simulink model "Drehteller"  (R2021a)
settings: Solver=VariableStepAuto  StartTime=0.0  StopTime=10.0  RelTol=1e-3
values from neighbouring files (symbols this model uses):
  A = 5    [Parametriesierung.m]
  I = 0.5    [Parametriesierung.m]
  igetr = 1080    [Parametriesierung.m]
  K = 8    [Parametriesierung.m]
  MRK = 1    [Parametriesierung.m]
  PHI = 0.001    [Parametriesierung.m]
  Ra = 40    [Parametriesierung.m]
  U = 24    [Parametriesierung.m]
settings Model: Creator=Oceaner  LastModifiedBy=Oceaner

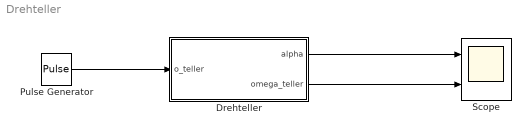
== system Drehteller ==
  Drehteller : Subsystem
  Pulse Generator : DiscretePulseGenerator  PulseType=Time based  PulseWidth=50
  Scope : Scope  NumInputPorts=2
  wires:
  Pulse Generator/1 -> Drehteller/1(o_teller)
  Drehteller/1(alpha) -> Scope/1
  Drehteller/2(omega_teller) -> Scope/2

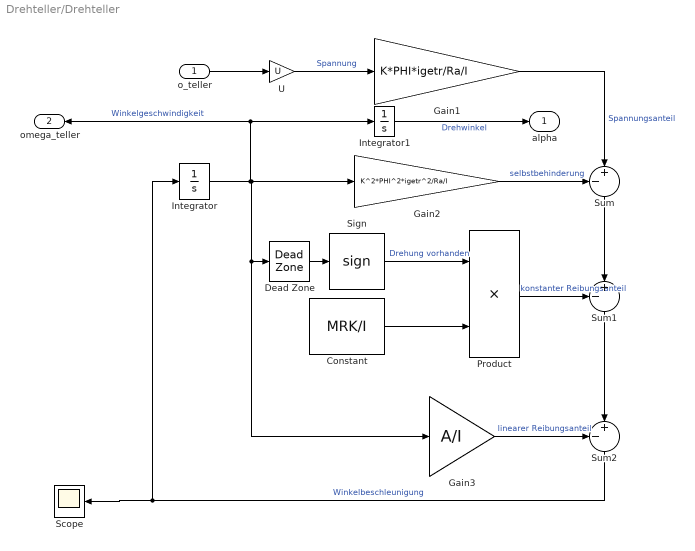
== system Drehteller/Drehteller ==
  o_teller : Inport
  Constant : Constant  Value=MRK/I
  Dead Zone : DeadZone  SaturateOnIntegerOverflow=on
  Gain1 : Gain  Gain=K*PHI*igetr/Ra/I
  Gain2 : Gain  Gain=K^2*PHI^2*igetr^2/Ra/I
  Gain3 : Gain  Gain=A/I
  Integrator : Integrator
  Integrator1 : Integrator
  Product : Product
  Scope : Scope
  Sign : Signum
  Sum : Sum  Inputs=-+|
  Sum1 : Sum  Inputs=-+|
  Sum2 : Sum  Inputs=-+|
  U : Gain  Gain=U
  alpha : Outport
  omega_teller : Outport  Port=2
  wires:
  U/1 -> Gain1/1  "Spannung"
  Product/1 -> Sum1/1  "konstanter Reibungsanteil"
  Integrator/1 -> Gain2/1, Gain3/1, Dead Zone/1, omega_teller/1, Integrator1/1  "Winkelgeschwindigkeit"
  Gain1/1 -> Sum/2  "Spannungsanteil"
  Sum1/1 -> Sum2/2
  Sum/1 -> Sum1/2
  o_teller/1 -> U/1
  Gain2/1 -> Sum/1  "selbstbehinderung"
  Sign/1 -> Product/1  "Drehung vorhanden"
  Dead Zone/1 -> Sign/1
  Gain3/1 -> Sum2/1  "linearer Reibungsanteil"
  Sum2/1 -> Scope/1, Integrator/1  "Winkelbeschleunigung"
  Constant/1 -> Product/2
  Integrator1/1 -> alpha/1  "Drehwinkel"
